simulink model "lift_parallel"  (R2020a)
settings: Solver=VariableStepAuto  StartTime=0.0  StopTime=10.0  RelTol=1e-3
settings Model: Creator=kiran  LastModifiedBy=kiran

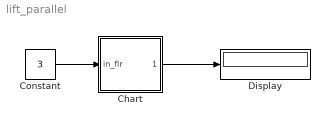
== system lift_parallel ==
  Chart : Stateflow chart  TreatAsAtomicUnit=on
  Constant : Constant  Value=3
  Display : Display
  wires:
  Constant/1 -> Chart/1(in_flr)
  Chart/1(out_flr) -> Display/1

== stateflow chart lift_parallel/Chart ==
  state Lift [parallel]
    settings: executionOrder=1
    state down
      during:
      crnt_flr=crnt_flr-1;
      out_flr=crnt_flr;
    state stop
      during:
      out_flr=crnt_flr
    state up
      during:
      crnt_flr=crnt_flr+1;
      out_flr=crnt_flr;
    (default) -> stop
    stop -> stop [order 3] : [crnt_flr==in_flr]
    up -> stop : [crnt_flr==in_flr]
    stop -> down [order 2] : [crnt_flr>in_flr]{send(down,floor_control)}
    down -> stop : [crnt_flr==in_flr]
    stop -> up [order 1] : [crnt_flr<in_flr]{send(up,floor_control)}
  state floor_control [parallel]
    settings: executionOrder=2
    state flr1
      en:
      crnt_flr=0;
      out_flr=1;
    state flr2
      en:
      out_flr=2;
    state flr3
      en:
      out_flr=3;
    state flr4
      en:
      out_flr=4;
    state flr5
      en:
      out_flr=5;
    (default) -> flr1
    flr1 -> flr2 [order 1] : up
    flr4 -> flr5 [order 1] : up
    flr2 -> flr3 [order 1] : up
    flr3 -> flr4 [order 1] : up
    flr2 -> flr1 [order 2] : down
    flr3 -> flr2 [order 2] : down
    flr4 -> flr3 [order 2] : down
    flr5 -> flr4 [order 1] : down
    flr1 -> flr1 [order 2] : down
    flr5 -> flr5 [order 2] : up
  data: in_flr input; out_flr output; crnt_flr local =0
  events: down local RISING_EDGE_EVENT; up local RISING_EDGE_EVENT
